simulink model "EPT"  (R2019b)
settings: Solver=FixedStepDiscrete  StartTime=0.0  StopTime=5  FixedStep=0.005  RelTol=1e-3  EnableMultiTasking=on
PreLoadFcn:
  | try, model_open; catch, disp('Error occurred while executing model pre-load callback: model_open.m'); disp('Please assure that the MATLAB working directory is set to the model directory before opening.'); end
InitFcn:
  | try, model_open; catch, end
undefined symbols (not defined in the file or in its folder): Bridge, GCM, H, ln, raptor_get_param_eval, raptor_get_safe_string, raptor_xcp_function
libraries: Raptor_lib x2810, simulink x374, hdlsllib x19
(part 22 of 45)

== system EPT/Foreground_TimeBase_5ms/CAN/CAN3_exec/SWCU/SWCU OP Status-G6 ==
  Trigger : TriggerPort  VariantControl=Variant  PortDimensions=1
  raptor_can_rxmsg : Raptor_lib/CAN/raptor_can_rxmsg  canDefinition=struct('dbcFile', 'EPTvsSWCU.dbc','message', 'SWCU_OP_Status_G6_SWUBP1','comment', '','signals', {{'SWCU_BPSWU_READY','SWCU_BPSWU_HV_ENABLED','SWCU_BPSWU_EW','SWCU_BPSWU_EW_CODE','SWCU_BPSWU_FCCAP','SWCU_BPSWU_RSOC','SWCU_BPSWU_CURR','SWCU_BPSWU_VOLT','SWCU_BPSWU_TEMP','SWCU_BPSWU_VCELL_MAX','SWCU_BPSWU_VCELL_MIN'}},'enabled', [ 1 1 1 1 1 1 1 1 1 1 1;],'canBus', '''CAN3''','messageID', [ 410055780;],'idMask', [ 536870911;],'payloadMask', [],'payloadValue', [],'period', [ 0;],'mailbox', '''''','queueSize', [ 1;],'label', [ 1;],'ver', [ 2;],'showID', [ 0;],'showRaw', [ 0;],'fill', [ 0;],'editID', [ 0;],'signalOrder', [ 2;])  canBus='CAN3'  mailbox=''  payloadMask=[]  payloadValue=[]  idMask=hex2dec('1FFFFFFF')  queueSize=1  showID=0  label=1  fill=0  id=410055780  showRaw=0  showAge=1  signalOrder=2  signalInfo={{struct('Name', 'SWCU_BPSWU_HV_ENABLED','Startbit', [ 0;],'SignalSize', [ 1;],'ByteOrder', 'LittleEndian','ValueType', 'UNSIGNED','Class', 'uint8','Signed', [ 0;],'Factor', [ 1;],'Offset', [ 0;],'Min', [ 0;],'Max', [ 0;],'Units', '','Comment', '','StartBit', [ 1;]),struct('Name', 'SWCU_BPSWU_EW_CODE','Startbit', [ 0;],'SignalSize', [ 5;],'ByteOrder', 'LittleEndian','ValueType', 'UNSIGNED','Class', 'uint8','Signed', [ 0;],'Factor', [ 1;],'Offset', [ 0;],'Min', [ 0;],'Max', [ 0;],'Units', '','Comment', '','StartBit', [ 3;]),struct('Name', 'SWCU_BPSWU_EW','Startbit', [ 0;],'SignalSize', [ 1;],'ByteOrder', 'LittleEndian','ValueType', 'UNSIGNED','Class', 'uint8','Signed', [ 0;],'Factor', [ 1;],'Offset', [ 0;],'Min', [ 0;],'Max', [ 0;],'Units', '','Comment', '','StartBit', [ 2;]),struct('Name', 'SWCU_BPSWU_VCELL_MIN','Startbit', [ 0;],'SignalSize', [ 8;],'ByteOrder', 'LittleEndian','ValueType', 'UNSIGNED','Class', 'uint8','Signed', [ 0;],'Factor', [ 0.01;],'Offset', [ 2;],'Min', [ 0;],'Max', [ 0;],'Units', 'V','Comment', '','StartBit', [ 56;]),struct('Name', 'SWCU_BPSWU_VCELL_MAX','Startbit', [ 0;],'SignalSize', [ 8;],'ByteOrder', 'LittleEndian','ValueType', 'UNSIGNED','Class', 'uint8','Signed', [ 0;],'Factor', [ 0.01;],'Offset', [ 2;],'Min', [ 0;],'Max', [ 0;],'Units', 'V','Comment', '','StartBit', [ 48;]),struct('Name', 'SWCU_BPSWU_VOLT','Startbit', [ 0;],'SignalSize', [ 8;],'ByteOrder', 'LittleEndian','ValueType', 'UNSIGNED','Class', 'uint8','Signed', [ 0;],'Factor', [ 1;],'Offset', [ 0;],'Min', [ 0;],'Max', [ 0;],'Units', 'V','Comment', '','StartBit', [ 32;]),struct('Name', 'SWCU_BPSWU_TEMP','Startbit', [ 0;],'SignalSize', [ 8;],'ByteOrder', 'LittleEndian','ValueType', 'UNSIGNED','Class', 'uint8','Signed', [ 0;],'Factor', [ 1;],'Offset', [ -40;],'Min', [ 0;],'Max', [ 0;],'Units', '℃','Comment', '','StartBit', [ 40;]),struct('Name', 'SWCU_BPSWU_RSOC','Startbit', [ 0;],'SignalSize', [ 8;],'ByteOrder', 'LittleEndian','ValueType', 'UNSIGNED','Class', 'uint8','Signed', [ 0;],'Factor', [ 0.5;],'Offset', [ -12.5;],'Min', [ 0;],'Max', [ 0;],'Units', '%','Comment', '','StartBit', [ 16;]),struct('Name', 'SWCU_BPSWU_CURR','Startbit', [ 0;],'SignalSize', [ 8;],'ByteOrder', 'LittleEndian','ValueType', 'UNSIGNED','Class', 'uint8','Signed', [ 0;],'Factor', [ 0.8;],'Offset', [ -100;],'Min', [ 0;],'Max', [ 0;],'Units', 'A','Comment', '','StartBit', [ 24;]),struct('Name', 'SWCU_BPSWU_FCCAP','Startbit', [ 0;],'SignalSize', [ 8;],'ByteOrder', 'LittleEndian','ValueType', 'UNSIGNED','Class', 'uint8','Signed', [ 0;],'Factor', [ 0.4;],'Offset', [ 0;],'Min', [ 0;],'Max', [ 0;],'Units', 'Ah','Comment', '','StartBit', [ 8;]),struct('Name', 'SWCU_BPSWU_READY','Startbit', [ 0;],'SignalSize', [ 1;],'ByteOrder', 'LittleEndian','ValueType', 'UNSIGNED','Class', 'uint8','Signed', [ 0;],'Factor', [ 1;],'Offset', [ 0;],'Min', [ 0;],'Max', [ 0;],'Units', '','Comment', '','StartBit', [ 0;])}}
      settings: SourceProductName=Raptor
  raptor_data_def : Raptor_lib/Data Storage/raptor_data_def  dataName='SWCU_BPSWU1_HV_ENABLED'  initValue=0  dataType=double  storage=Calibration  calVisible=on  calType=Measurement  calDispType=Number  calEnum={'False', 'True'}  calGain=1.0  calOffset=0  calMin=-inf  calMax=inf  calFormat='-1'  calUnit=''  calHelp=''  calAccess=1  calFunction=raptor_xcp_function(gcb)  calDispHeaders=off  calColHeaders={'Col1' 'Col2' 'Col3'}  calRowHeaders={'Row1' 'Row2' 'Row3'}
      settings: SourceProductName=Raptor
  raptor_data_def1 : Raptor_lib/Data Storage/raptor_data_def  dataName='SWCU_BPSWU1_READY'  initValue=0  dataType=double  storage=Calibration  calVisible=on  calType=Measurement  calDispType=Number  calEnum={'False', 'True'}  calGain=1.0  calOffset=0  calMin=-inf  calMax=inf  calFormat='-1'  calUnit=''  calHelp=''  calAccess=1  calFunction=raptor_xcp_function(gcb)  calDispHeaders=off  calColHeaders={'Col1' 'Col2' 'Col3'}  calRowHeaders={'Row1' 'Row2' 'Row3'}
      settings: SourceProductName=Raptor
  raptor_data_def10 : Raptor_lib/Data Storage/raptor_data_def  dataName='SWCU_BPSWU1_VCELL_MAX'  initValue=0  dataType=double  storage=Calibration  calVisible=on  calType=Measurement  calDispType=Number  calEnum={'False', 'True'}  calGain=1.0  calOffset=0  calMin=-inf  calMax=inf  calFormat='-1'  calUnit=''  calHelp=''  calAccess=1  calFunction=raptor_xcp_function(gcb)  calDispHeaders=off  calColHeaders={'Col1' 'Col2' 'Col3'}  calRowHeaders={'Row1' 'Row2' 'Row3'}
      settings: SourceProductName=Raptor
  raptor_data_def2 : Raptor_lib/Data Storage/raptor_data_def  dataName='SWCU_BPSWU1_EW'  initValue=0  dataType=double  storage=Calibration  calVisible=on  calType=Measurement  calDispType=Number  calEnum={'False', 'True'}  calGain=1.0  calOffset=0  calMin=-inf  calMax=inf  calFormat='-1'  calUnit=''  calHelp=''  calAccess=1  calFunction=raptor_xcp_function(gcb)  calDispHeaders=off  calColHeaders={'Col1' 'Col2' 'Col3'}  calRowHeaders={'Row1' 'Row2' 'Row3'}
      settings: SourceProductName=Raptor
  raptor_data_def3 : Raptor_lib/Data Storage/raptor_data_def  dataName='SWCU_BPSWU1_FCCAP'  initValue=0  dataType=double  storage=Calibration  calVisible=on  calType=Measurement  calDispType=Number  calEnum={'False', 'True'}  calGain=1.0  calOffset=0  calMin=-inf  calMax=inf  calFormat='-1'  calUnit=''  calHelp=''  calAccess=1  calFunction=raptor_xcp_function(gcb)  calDispHeaders=off  calColHeaders={'Col1' 'Col2' 'Col3'}  calRowHeaders={'Row1' 'Row2' 'Row3'}
      settings: SourceProductName=Raptor
  raptor_data_def4 : Raptor_lib/Data Storage/raptor_data_def  dataName='SWCU_BPSWU1_RSOC'  initValue=0  dataType=double  storage=Calibration  calVisible=on  calType=Measurement  calDispType=Number  calEnum={'False', 'True'}  calGain=1.0  calOffset=0  calMin=-inf  calMax=inf  calFormat='-1'  calUnit=''  calHelp=''  calAccess=1  calFunction=raptor_xcp_function(gcb)  calDispHeaders=off  calColHeaders={'Col1' 'Col2' 'Col3'}  calRowHeaders={'Row1' 'Row2' 'Row3'}
      settings: SourceProductName=Raptor
  raptor_data_def5 : Raptor_lib/Data Storage/raptor_data_def  dataName='SWCU_BPSWU1_EW_CODE'  initValue=0  dataType=double  storage=Calibration  calVisible=on  calType=Measurement  calDispType=Number  calEnum={'False', 'True'}  calGain=1.0  calOffset=0  calMin=-inf  calMax=inf  calFormat='-1'  calUnit=''  calHelp=''  calAccess=1  calFunction=raptor_xcp_function(gcb)  calDispHeaders=off  calColHeaders={'Col1' 'Col2' 'Col3'}  calRowHeaders={'Row1' 'Row2' 'Row3'}
      settings: SourceProductName=Raptor
  raptor_data_def6 : Raptor_lib/Data Storage/raptor_data_def  dataName='SWCU_BPSWU1_CURR'  initValue=0  dataType=double  storage=Calibration  calVisible=on  calType=Measurement  calDispType=Number  calEnum={'False', 'True'}  calGain=1.0  calOffset=0  calMin=-inf  calMax=inf  calFormat='-1'  calUnit=''  calHelp=''  calAccess=1  calFunction=raptor_xcp_function(gcb)  calDispHeaders=off  calColHeaders={'Col1' 'Col2' 'Col3'}  calRowHeaders={'Row1' 'Row2' 'Row3'}
      settings: SourceProductName=Raptor
  raptor_data_def7 : Raptor_lib/Data Storage/raptor_data_def  dataName='SWCU_BPSWU1_TEMP'  initValue=0  dataType=double  storage=Calibration  calVisible=on  calType=Measurement  calDispType=Number  calEnum={'False', 'True'}  calGain=1.0  calOffset=0  calMin=-inf  calMax=inf  calFormat='-1'  calUnit=''  calHelp=''  calAccess=1  calFunction=raptor_xcp_function(gcb)  calDispHeaders=off  calColHeaders={'Col1' 'Col2' 'Col3'}  calRowHeaders={'Row1' 'Row2' 'Row3'}
      settings: SourceProductName=Raptor
  raptor_data_def8 : Raptor_lib/Data Storage/raptor_data_def  dataName='SWCU_BPSWU1_VCELL_MIN'  initValue=0  dataType=double  storage=Calibration  calVisible=on  calType=Measurement  calDispType=Number  calEnum={'False', 'True'}  calGain=1.0  calOffset=0  calMin=-inf  calMax=inf  calFormat='-1'  calUnit=''  calHelp=''  calAccess=1  calFunction=raptor_xcp_function(gcb)  calDispHeaders=off  calColHeaders={'Col1' 'Col2' 'Col3'}  calRowHeaders={'Row1' 'Row2' 'Row3'}
      settings: SourceProductName=Raptor
  raptor_data_def9 : Raptor_lib/Data Storage/raptor_data_def  dataName='SWCU_BPSWU1_VOLT'  initValue=0  dataType=double  storage=Calibration  calVisible=on  calType=Measurement  calDispType=Number  calEnum={'False', 'True'}  calGain=1.0  calOffset=0  calMin=-inf  calMax=inf  calFormat='-1'  calUnit=''  calHelp=''  calAccess=1  calFunction=raptor_xcp_function(gcb)  calDispHeaders=off  calColHeaders={'Col1' 'Col2' 'Col3'}  calRowHeaders={'Row1' 'Row2' 'Row3'}
      settings: SourceProductName=Raptor
  raptor_data_write : Raptor_lib/Data Storage/raptor_data_write  dataName='SWCU_BPSWU1_HV_ENABLED'  dataShape=Scalar  idxSource=Input Port  idxRow=1  idxCol=1
      settings: SourceProductName=Raptor
  raptor_data_write1 : Raptor_lib/Data Storage/raptor_data_write  dataName='SWCU_BPSWU1_READY'  dataShape=Scalar  idxSource=Input Port  idxRow=1  idxCol=1
      settings: SourceProductName=Raptor
  raptor_data_write10 : Raptor_lib/Data Storage/raptor_data_write  dataName='SWCU_BPSWU1_VCELL_MIN'  dataShape=Scalar  idxSource=Input Port  idxRow=1  idxCol=1
      settings: SourceProductName=Raptor
  raptor_data_write2 : Raptor_lib/Data Storage/raptor_data_write  dataName='SWCU_BPSWU1_EW'  dataShape=Scalar  idxSource=Input Port  idxRow=1  idxCol=1
      settings: SourceProductName=Raptor
  raptor_data_write3 : Raptor_lib/Data Storage/raptor_data_write  dataName='SWCU_BPSWU1_EW_CODE'  dataShape=Scalar  idxSource=Input Port  idxRow=1  idxCol=1
      settings: SourceProductName=Raptor
  raptor_data_write4 : Raptor_lib/Data Storage/raptor_data_write  dataName='SWCU_BPSWU1_RSOC'  dataShape=Scalar  idxSource=Input Port  idxRow=1  idxCol=1
      settings: SourceProductName=Raptor
  raptor_data_write5 : Raptor_lib/Data Storage/raptor_data_write  dataName='SWCU_BPSWU1_FCCAP'  dataShape=Scalar  idxSource=Input Port  idxRow=1  idxCol=1
      settings: SourceProductName=Raptor
  raptor_data_write6 : Raptor_lib/Data Storage/raptor_data_write  dataName='SWCU_BPSWU1_CURR'  dataShape=Scalar  idxSource=Input Port  idxRow=1  idxCol=1
      settings: SourceProductName=Raptor
  raptor_data_write7 : Raptor_lib/Data Storage/raptor_data_write  dataName='SWCU_BPSWU1_VOLT'  dataShape=Scalar  idxSource=Input Port  idxRow=1  idxCol=1
      settings: SourceProductName=Raptor
  raptor_data_write8 : Raptor_lib/Data Storage/raptor_data_write  dataName='SWCU_BPSWU1_TEMP'  dataShape=Scalar  idxSource=Input Port  idxRow=1  idxCol=1
      settings: SourceProductName=Raptor
  raptor_data_write9 : Raptor_lib/Data Storage/raptor_data_write  dataName='SWCU_BPSWU1_VCELL_MAX'  dataShape=Scalar  idxSource=Input Port  idxRow=1  idxCol=1
      settings: SourceProductName=Raptor
  wires:
  raptor_can_rxmsg/3 -> raptor_data_write/1  "SWCU_BPSWU_HV_ENABLED"
  raptor_can_rxmsg/2 -> raptor_data_write1/1  "SWCU_BPSWU_READY"
  raptor_can_rxmsg/4 -> raptor_data_write2/1  "SWCU_BPSWU_EW"
  raptor_can_rxmsg/5 -> raptor_data_write3/1  "SWCU_BPSWU_EW_CODE"
  raptor_can_rxmsg/9 -> raptor_data_write7/1  "SWCU_BPSWU_VOLT"
  raptor_can_rxmsg/8 -> raptor_data_write6/1  "SWCU_BPSWU_CURR"
  raptor_can_rxmsg/6 -> raptor_data_write5/1  "SWCU_BPSWU_FCCAP"
  raptor_can_rxmsg/7 -> raptor_data_write4/1  "SWCU_BPSWU_RSOC"
  raptor_can_rxmsg/10 -> raptor_data_write8/1  "SWCU_BPSWU_TEMP"
  raptor_can_rxmsg/11 -> raptor_data_write9/1  "SWCU_BPSWU_VCELL_MAX"
  raptor_can_rxmsg/12 -> raptor_data_write10/1  "SWCU_BPSWU_VCELL_MIN"

== system EPT/Foreground_TimeBase_5ms/CAN/CAN3_exec/SWCU/SWCU OP Status-G7 ==
  Trigger : TriggerPort  VariantControl=Variant  PortDimensions=1
  raptor_can_rxmsg : Raptor_lib/CAN/raptor_can_rxmsg  canDefinition=struct('dbcFile', 'EPTvsSWCU.dbc','message', 'SWCU_OP_Status_G7_SWUBP2','comment', '','signals', {{'SWCU_BPSWU_READY','SWCU_BPSWU_HV_ENABLED','SWCU_BPSWU_EW','SWCU_BPSWU_EW_CODE','SWCU_BPSWU_FCCAP','SWCU_BPSWU_RSOC','SWCU_BPSWU_CURR','SWCU_BPSWU_VOLT','SWCU_BPSWU_TEMP','SWCU_BPSWU_VCELL_MAX','SWCU_BPSWU_VCELL_MIN'}},'enabled', [ 1 1 1 1 1 1 1 1 1 1 1;],'canBus', '''CAN3''','messageID', [ 410121316;],'idMask', [ 536870911;],'payloadMask', [],'payloadValue', [],'period', [ 0;],'mailbox', '''''','queueSize', [ 1;],'label', [ 0;],'ver', [ 2;],'showID', [ 0;],'showRaw', [ 0;],'fill', [ 0;],'editID', [ 0;],'signalOrder', [ 2;])  canBus='CAN3'  mailbox=''  payloadMask=[]  payloadValue=[]  idMask=hex2dec('1FFFFFFF')  queueSize=1  showID=0  label=0  fill=0  id=410121316  showRaw=0  showAge=1  signalOrder=2  signalInfo={{struct('Name', 'SWCU_BPSWU_HV_ENABLED','Startbit', [ 0;],'SignalSize', [ 1;],'ByteOrder', 'LittleEndian','ValueType', 'UNSIGNED','Class', 'uint8','Signed', [ 0;],'Factor', [ 1;],'Offset', [ 0;],'Min', [ 0;],'Max', [ 0;],'Units', '','Comment', '','StartBit', [ 1;]),struct('Name', 'SWCU_BPSWU_EW_CODE','Startbit', [ 0;],'SignalSize', [ 5;],'ByteOrder', 'LittleEndian','ValueType', 'UNSIGNED','Class', 'uint8','Signed', [ 0;],'Factor', [ 1;],'Offset', [ 0;],'Min', [ 0;],'Max', [ 0;],'Units', '','Comment', '','StartBit', [ 3;]),struct('Name', 'SWCU_BPSWU_EW','Startbit', [ 0;],'SignalSize', [ 1;],'ByteOrder', 'LittleEndian','ValueType', 'UNSIGNED','Class', 'uint8','Signed', [ 0;],'Factor', [ 1;],'Offset', [ 0;],'Min', [ 0;],'Max', [ 0;],'Units', '','Comment', '','StartBit', [ 2;]),struct('Name', 'SWCU_BPSWU_VCELL_MIN','Startbit', [ 0;],'SignalSize', [ 8;],'ByteOrder', 'LittleEndian','ValueType', 'UNSIGNED','Class', 'uint8','Signed', [ 0;],'Factor', [ 0.01;],'Offset', [ 2;],'Min', [ 0;],'Max', [ 0;],'Units', 'V','Comment', '','StartBit', [ 56;]),struct('Name', 'SWCU_BPSWU_VCELL_MAX','Startbit', [ 0;],'SignalSize', [ 8;],'ByteOrder', 'LittleEndian','ValueType', 'UNSIGNED','Class', 'uint8','Signed', [ 0;],'Factor', [ 0.01;],'Offset', [ 2;],'Min', [ 0;],'Max', [ 0;],'Units', 'V','Comment', '','StartBit', [ 48;]),struct('Name', 'SWCU_BPSWU_VOLT','Startbit', [ 0;],'SignalSize', [ 8;],'ByteOrder', 'LittleEndian','ValueType', 'UNSIGNED','Class', 'uint8','Signed', [ 0;],'Factor', [ 1;],'Offset', [ 0;],'Min', [ 0;],'Max', [ 0;],'Units', 'V','Comment', '','StartBit', [ 32;]),struct('Name', 'SWCU_BPSWU_TEMP','Startbit', [ 0;],'SignalSize', [ 8;],'ByteOrder', 'LittleEndian','ValueType', 'UNSIGNED','Class', 'uint8','Signed', [ 0;],'Factor', [ 1;],'Offset', [ -40;],'Min', [ 0;],'Max', [ 0;],'Units', '℃','Comment', '','StartBit', [ 40;]),struct('Name', 'SWCU_BPSWU_RSOC','Startbit', [ 0;],'SignalSize', [ 8;],'ByteOrder', 'LittleEndian','ValueType', 'UNSIGNED','Class', 'uint8','Signed', [ 0;],'Factor', [ 0.5;],'Offset', [ -12.5;],'Min', [ 0;],'Max', [ 0;],'Units', '%','Comment', '','StartBit', [ 16;]),struct('Name', 'SWCU_BPSWU_CURR','Startbit', [ 0;],'SignalSize', [ 8;],'ByteOrder', 'LittleEndian','ValueType', 'UNSIGNED','Class', 'uint8','Signed', [ 0;],'Factor', [ 0.8;],'Offset', [ -100;],'Min', [ 0;],'Max', [ 0;],'Units', 'A','Comment', '','StartBit', [ 24;]),struct('Name', 'SWCU_BPSWU_FCCAP','Startbit', [ 0;],'SignalSize', [ 8;],'ByteOrder', 'LittleEndian','ValueType', 'UNSIGNED','Class', 'uint8','Signed', [ 0;],'Factor', [ 0.4;],'Offset', [ 0;],'Min', [ 0;],'Max', [ 0;],'Units', 'Ah','Comment', '','StartBit', [ 8;]),struct('Name', 'SWCU_BPSWU_READY','Startbit', [ 0;],'SignalSize', [ 1;],'ByteOrder', 'LittleEndian','ValueType', 'UNSIGNED','Class', 'uint8','Signed', [ 0;],'Factor', [ 1;],'Offset', [ 0;],'Min', [ 0;],'Max', [ 0;],'Units', '','Comment', '','StartBit', [ 0;])}}
      settings: SourceProductName=Raptor
  raptor_data_def : Raptor_lib/Data Storage/raptor_data_def  dataName='SWCU_BPSWU2_HV_ENABLED'  initValue=0  dataType=double  storage=Calibration  calVisible=on  calType=Measurement  calDispType=Number  calEnum={'False', 'True'}  calGain=1.0  calOffset=0  calMin=-inf  calMax=inf  calFormat='-1'  calUnit=''  calHelp=''  calAccess=1  calFunction=raptor_xcp_function(gcb)  calDispHeaders=off  calColHeaders={'Col1' 'Col2' 'Col3'}  calRowHeaders={'Row1' 'Row2' 'Row3'}
      settings: SourceProductName=Raptor
  raptor_data_def1 : Raptor_lib/Data Storage/raptor_data_def  dataName='SWCU_BPSWU2_READY'  initValue=0  dataType=double  storage=Calibration  calVisible=on  calType=Measurement  calDispType=Number  calEnum={'False', 'True'}  calGain=1.0  calOffset=0  calMin=-inf  calMax=inf  calFormat='-1'  calUnit=''  calHelp=''  calAccess=1  calFunction=raptor_xcp_function(gcb)  calDispHeaders=off  calColHeaders={'Col1' 'Col2' 'Col3'}  calRowHeaders={'Row1' 'Row2' 'Row3'}
      settings: SourceProductName=Raptor
  raptor_data_def10 : Raptor_lib/Data Storage/raptor_data_def  dataName='SWCU_BPSWU2_VCELL_MAX'  initValue=0  dataType=double  storage=Calibration  calVisible=on  calType=Measurement  calDispType=Number  calEnum={'False', 'True'}  calGain=1.0  calOffset=0  calMin=-inf  calMax=inf  calFormat='-1'  calUnit=''  calHelp=''  calAccess=1  calFunction=raptor_xcp_function(gcb)  calDispHeaders=off  calColHeaders={'Col1' 'Col2' 'Col3'}  calRowHeaders={'Row1' 'Row2' 'Row3'}
      settings: SourceProductName=Raptor
  raptor_data_def2 : Raptor_lib/Data Storage/raptor_data_def  dataName='SWCU_BPSWU2_EW'  initValue=0  dataType=double  storage=Calibration  calVisible=on  calType=Measurement  calDispType=Number  calEnum={'False', 'True'}  calGain=1.0  calOffset=0  calMin=-inf  calMax=inf  calFormat='-1'  calUnit=''  calHelp=''  calAccess=1  calFunction=raptor_xcp_function(gcb)  calDispHeaders=off  calColHeaders={'Col1' 'Col2' 'Col3'}  calRowHeaders={'Row1' 'Row2' 'Row3'}
      settings: SourceProductName=Raptor
  raptor_data_def3 : Raptor_lib/Data Storage/raptor_data_def  dataName='SWCU_BPSWU2_FCCAP'  initValue=0  dataType=double  storage=Calibration  calVisible=on  calType=Measurement  calDispType=Number  calEnum={'False', 'True'}  calGain=1.0  calOffset=0  calMin=-inf  calMax=inf  calFormat='-1'  calUnit=''  calHelp=''  calAccess=1  calFunction=raptor_xcp_function(gcb)  calDispHeaders=off  calColHeaders={'Col1' 'Col2' 'Col3'}  calRowHeaders={'Row1' 'Row2' 'Row3'}
      settings: SourceProductName=Raptor
  raptor_data_def4 : Raptor_lib/Data Storage/raptor_data_def  dataName='SWCU_BPSWU2_RSOC'  initValue=0  dataType=double  storage=Calibration  calVisible=on  calType=Measurement  calDispType=Number  calEnum={'False', 'True'}  calGain=1.0  calOffset=0  calMin=-inf  calMax=inf  calFormat='-1'  calUnit=''  calHelp=''  calAccess=1  calFunction=raptor_xcp_function(gcb)  calDispHeaders=off  calColHeaders={'Col1' 'Col2' 'Col3'}  calRowHeaders={'Row1' 'Row2' 'Row3'}
      settings: SourceProductName=Raptor
  raptor_data_def5 : Raptor_lib/Data Storage/raptor_data_def  dataName='SWCU_BPSWU2_EW_CODE'  initValue=0  dataType=double  storage=Calibration  calVisible=on  calType=Measurement  calDispType=Number  calEnum={'False', 'True'}  calGain=1.0  calOffset=0  calMin=-inf  calMax=inf  calFormat='-1'  calUnit=''  calHelp=''  calAccess=1  calFunction=raptor_xcp_function(gcb)  calDispHeaders=off  calColHeaders={'Col1' 'Col2' 'Col3'}  calRowHeaders={'Row1' 'Row2' 'Row3'}
      settings: SourceProductName=Raptor
  raptor_data_def6 : Raptor_lib/Data Storage/raptor_data_def  dataName='SWCU_BPSWU2_CURR'  initValue=0  dataType=double  storage=Calibration  calVisible=on  calType=Measurement  calDispType=Number  calEnum={'False', 'True'}  calGain=1.0  calOffset=0  calMin=-inf  calMax=inf  calFormat='-1'  calUnit=''  calHelp=''  calAccess=1  calFunction=raptor_xcp_function(gcb)  calDispHeaders=off  calColHeaders={'Col1' 'Col2' 'Col3'}  calRowHeaders={'Row1' 'Row2' 'Row3'}
      settings: SourceProductName=Raptor
  raptor_data_def7 : Raptor_lib/Data Storage/raptor_data_def  dataName='SWCU_BPSWU2_TEMP'  initValue=0  dataType=double  storage=Calibration  calVisible=on  calType=Measurement  calDispType=Number  calEnum={'False', 'True'}  calGain=1.0  calOffset=0  calMin=-inf  calMax=inf  calFormat='-1'  calUnit=''  calHelp=''  calAccess=1  calFunction=raptor_xcp_function(gcb)  calDispHeaders=off  calColHeaders={'Col1' 'Col2' 'Col3'}  calRowHeaders={'Row1' 'Row2' 'Row3'}
      settings: SourceProductName=Raptor
  raptor_data_def8 : Raptor_lib/Data Storage/raptor_data_def  dataName='SWCU_BPSWU2_VCELL_MIN'  initValue=0  dataType=double  storage=Calibration  calVisible=on  calType=Measurement  calDispType=Number  calEnum={'False', 'True'}  calGain=1.0  calOffset=0  calMin=-inf  calMax=inf  calFormat='-1'  calUnit=''  calHelp=''  calAccess=1  calFunction=raptor_xcp_function(gcb)  calDispHeaders=off  calColHeaders={'Col1' 'Col2' 'Col3'}  calRowHeaders={'Row1' 'Row2' 'Row3'}
      settings: SourceProductName=Raptor
  raptor_data_def9 : Raptor_lib/Data Storage/raptor_data_def  dataName='SWCU_BPSWU2_VOLT'  initValue=0  dataType=double  storage=Calibration  calVisible=on  calType=Measurement  calDispType=Number  calEnum={'False', 'True'}  calGain=1.0  calOffset=0  calMin=-inf  calMax=inf  calFormat='-1'  calUnit=''  calHelp=''  calAccess=1  calFunction=raptor_xcp_function(gcb)  calDispHeaders=off  calColHeaders={'Col1' 'Col2' 'Col3'}  calRowHeaders={'Row1' 'Row2' 'Row3'}
      settings: SourceProductName=Raptor
  raptor_data_write : Raptor_lib/Data Storage/raptor_data_write  dataName='SWCU_BPSWU2_HV_ENABLED'  dataShape=Scalar  idxSource=Input Port  idxRow=1  idxCol=1
      settings: SourceProductName=Raptor
  raptor_data_write1 : Raptor_lib/Data Storage/raptor_data_write  dataName='SWCU_BPSWU2_READY'  dataShape=Scalar  idxSource=Input Port  idxRow=1  idxCol=1
      settings: SourceProductName=Raptor
  raptor_data_write10 : Raptor_lib/Data Storage/raptor_data_write  dataName='SWCU_BPSWU2_VCELL_MIN'  dataShape=Scalar  idxSource=Input Port  idxRow=1  idxCol=1
      settings: SourceProductName=Raptor
  raptor_data_write2 : Raptor_lib/Data Storage/raptor_data_write  dataName='SWCU_BPSWU2_EW'  dataShape=Scalar  idxSource=Input Port  idxRow=1  idxCol=1
      settings: SourceProductName=Raptor
  raptor_data_write3 : Raptor_lib/Data Storage/raptor_data_write  dataName='SWCU_BPSWU2_EW_CODE'  dataShape=Scalar  idxSource=Input Port  idxRow=1  idxCol=1
      settings: SourceProductName=Raptor
  raptor_data_write4 : Raptor_lib/Data Storage/raptor_data_write  dataName='SWCU_BPSWU2_RSOC'  dataShape=Scalar  idxSource=Input Port  idxRow=1  idxCol=1
      settings: SourceProductName=Raptor
  raptor_data_write5 : Raptor_lib/Data Storage/raptor_data_write  dataName='SWCU_BPSWU2_FCCAP'  dataShape=Scalar  idxSource=Input Port  idxRow=1  idxCol=1
      settings: SourceProductName=Raptor
  raptor_data_write6 : Raptor_lib/Data Storage/raptor_data_write  dataName='SWCU_BPSWU2_CURR'  dataShape=Scalar  idxSource=Input Port  idxRow=1  idxCol=1
      settings: SourceProductName=Raptor
  raptor_data_write7 : Raptor_lib/Data Storage/raptor_data_write  dataName='SWCU_BPSWU2_VOLT'  dataShape=Scalar  idxSource=Input Port  idxRow=1  idxCol=1
      settings: SourceProductName=Raptor
  raptor_data_write8 : Raptor_lib/Data Storage/raptor_data_write  dataName='SWCU_BPSWU2_TEMP'  dataShape=Scalar  idxSource=Input Port  idxRow=1  idxCol=1
      settings: SourceProductName=Raptor
  raptor_data_write9 : Raptor_lib/Data Storage/raptor_data_write  dataName='SWCU_BPSWU2_VCELL_MAX'  dataShape=Scalar  idxSource=Input Port  idxRow=1  idxCol=1
      settings: SourceProductName=Raptor
  wires:
  raptor_can_rxmsg/3 -> raptor_data_write/1  "SWCU_BPSWU_HV_ENABLED"
  raptor_can_rxmsg/8 -> raptor_data_write6/1  "SWCU_BPSWU_CURR"
  raptor_can_rxmsg/6 -> raptor_data_write5/1  "SWCU_BPSWU_FCCAP"
  raptor_can_rxmsg/9 -> raptor_data_write7/1  "SWCU_BPSWU_VOLT"
  raptor_can_rxmsg/7 -> raptor_data_write4/1  "SWCU_BPSWU_RSOC"
  raptor_can_rxmsg/5 -> raptor_data_write3/1  "SWCU_BPSWU_EW_CODE"
  raptor_can_rxmsg/4 -> raptor_data_write2/1  "SWCU_BPSWU_EW"
  raptor_can_rxmsg/11 -> raptor_data_write9/1  "SWCU_BPSWU_VCELL_MAX"
  raptor_can_rxmsg/12 -> raptor_data_write10/1  "SWCU_BPSWU_VCELL_MIN"
  raptor_can_rxmsg/2 -> raptor_data_write1/1  "SWCU_BPSWU_READY"
  raptor_can_rxmsg/10 -> raptor_data_write8/1  "SWCU_BPSWU_TEMP"

== system EPT/Foreground_TimeBase_5ms/CAN/CAN3_exec/SWCU/SWCU OP Status-G8 ==
  Trigger : TriggerPort  VariantControl=Variant  PortDimensions=1
  raptor_can_rxmsg : Raptor_lib/CAN/raptor_can_rxmsg  canDefinition=struct('dbcFile', 'EPTvsSWCU.dbc','message', 'SWCU_OP_Status_G8_SWUBP3','comment', '','signals', {{'SWCU_BPSWU_READY','SWCU_BPSWU_HV_ENABLED','SWCU_BPSWU_EW','SWCU_BPSWU_EW_CODE','SWCU_BPSWU_FCCAP','SWCU_BPSWU_RSOC','SWCU_BPSWU_CURR','SWCU_BPSWU_VOLT','SWCU_BPSWU_TEMP','SWCU_BPSWU_VCELL_MAX','SWCU_BPSWU_VCELL_MIN'}},'enabled', [ 1 1 1 1 1 1 1 1 1 1 1;],'canBus', '''CAN3''','messageID', [ 410186852;],'idMask', [ 536870911;],'payloadMask', [],'payloadValue', [],'period', [ 0;],'mailbox', '''''','queueSize', [ 1;],'label', [ 0;],'ver', [ 2;],'showID', [ 0;],'showRaw', [ 0;],'fill', [ 0;],'editID', [ 0;],'signalOrder', [ 2;])  canBus='CAN3'  mailbox=''  payloadMask=[]  payloadValue=[]  idMask=hex2dec('1FFFFFFF')  queueSize=1  showID=0  label=0  fill=0  id=410186852  showRaw=0  showAge=1  signalOrder=2  signalInfo={{struct('Name', 'SWCU_BPSWU_HV_ENABLED','Startbit', [ 0;],'SignalSize', [ 1;],'ByteOrder', 'LittleEndian','ValueType', 'UNSIGNED','Class', 'uint8','Signed', [ 0;],'Factor', [ 1;],'Offset', [ 0;],'Min', [ 0;],'Max', [ 0;],'Units', '','Comment', '','StartBit', [ 1;]),struct('Name', 'SWCU_BPSWU_EW_CODE','Startbit', [ 0;],'SignalSize', [ 5;],'ByteOrder', 'LittleEndian','ValueType', 'UNSIGNED','Class', 'uint8','Signed', [ 0;],'Factor', [ 1;],'Offset', [ 0;],'Min', [ 0;],'Max', [ 0;],'Units', '','Comment', '','StartBit', [ 3;]),struct('Name', 'SWCU_BPSWU_EW','Startbit', [ 0;],'SignalSize', [ 1;],'ByteOrder', 'LittleEndian','ValueType', 'UNSIGNED','Class', 'uint8','Signed', [ 0;],'Factor', [ 1;],'Offset', [ 0;],'Min', [ 0;],'Max', [ 0;],'Units', '','Comment', '','StartBit', [ 2;]),struct('Name', 'SWCU_BPSWU_VCELL_MIN','Startbit', [ 0;],'SignalSize', [ 8;],'ByteOrder', 'LittleEndian','ValueType', 'UNSIGNED','Class', 'uint8','Signed', [ 0;],'Factor', [ 0.01;],'Offset', [ 2;],'Min', [ 0;],'Max', [ 0;],'Units', 'V','Comment', '','StartBit', [ 56;]),struct('Name', 'SWCU_BPSWU_VCELL_MAX','Startbit', [ 0;],'SignalSize', [ 8;],'ByteOrder', 'LittleEndian','ValueType', 'UNSIGNED','Class', 'uint8','Signed', [ 0;],'Factor', [ 0.01;],'Offset', [ 2;],'Min', [ 0;],'Max', [ 0;],'Units', 'V','Comment', '','StartBit', [ 48;]),struct('Name', 'SWCU_BPSWU_VOLT','Startbit', [ 0;],'SignalSize', [ 8;],'ByteOrder', 'LittleEndian','ValueType', 'UNSIGNED','Class', 'uint8','Signed', [ 0;],'Factor', [ 1;],'Offset', [ 0;],'Min', [ 0;],'Max', [ 0;],'Units', 'V','Comment', '','StartBit', [ 32;]),struct('Name', 'SWCU_BPSWU_TEMP','Startbit', [ 0;],'SignalSize', [ 8;],'ByteOrder', 'LittleEndian','ValueType', 'UNSIGNED','Class', 'uint8','Signed', [ 0;],'Factor', [ 1;],'Offset', [ -40;],'Min', [ 0;],'Max', [ 0;],'Units', '℃','Comment', '','StartBit', [ 40;]),struct('Name', 'SWCU_BPSWU_RSOC','Startbit', [ 0;],'SignalSize', [ 8;],'ByteOrder', 'LittleEndian','ValueType', 'UNSIGNED','Class', 'uint8','Signed', [ 0;],'Factor', [ 0.5;],'Offset', [ -12.5;],'Min', [ 0;],'Max', [ 0;],'Units', '%','Comment', '','StartBit', [ 16;]),struct('Name', 'SWCU_BPSWU_CURR','Startbit', [ 0;],'SignalSize', [ 8;],'ByteOrder', 'LittleEndian','ValueType', 'UNSIGNED','Class', 'uint8','Signed', [ 0;],'Factor', [ 0.8;],'Offset', [ -100;],'Min', [ 0;],'Max', [ 0;],'Units', 'A','Comment', '','StartBit', [ 24;]),struct('Name', 'SWCU_BPSWU_FCCAP','Startbit', [ 0;],'SignalSize', [ 8;],'ByteOrder', 'LittleEndian','ValueType', 'UNSIGNED','Class', 'uint8','Signed', [ 0;],'Factor', [ 0.4;],'Offset', [ 0;],'Min', [ 0;],'Max', [ 0;],'Units', 'Ah','Comment', '','StartBit', [ 8;]),struct('Name', 'SWCU_BPSWU_READY','Startbit', [ 0;],'SignalSize', [ 1;],'ByteOrder', 'LittleEndian','ValueType', 'UNSIGNED','Class', 'uint8','Signed', [ 0;],'Factor', [ 1;],'Offset', [ 0;],'Min', [ 0;],'Max', [ 0;],'Units', '','Comment', '','StartBit', [ 0;])}}
      settings: SourceProductName=Raptor
  raptor_data_def : Raptor_lib/Data Storage/raptor_data_def  dataName='SWCU_BPSWU3_HV_ENABLED'  initValue=0  dataType=double  storage=Calibration  calVisible=on  calType=Measurement  calDispType=Number  calEnum={'False', 'True'}  calGain=1.0  calOffset=0  calMin=-inf  calMax=inf  calFormat='-1'  calUnit=''  calHelp=''  calAccess=1  calFunction=raptor_xcp_function(gcb)  calDispHeaders=off  calColHeaders={'Col1' 'Col2' 'Col3'}  calRowHeaders={'Row1' 'Row2' 'Row3'}
      settings: SourceProductName=Raptor
  raptor_data_def1 : Raptor_lib/Data Storage/raptor_data_def  dataName='SWCU_BPSWU3_READY'  initValue=0  dataType=double  storage=Calibration  calVisible=on  calType=Measurement  calDispType=Number  calEnum={'False', 'True'}  calGain=1.0  calOffset=0  calMin=-inf  calMax=inf  calFormat='-1'  calUnit=''  calHelp=''  calAccess=1  calFunction=raptor_xcp_function(gcb)  calDispHeaders=off  calColHeaders={'Col1' 'Col2' 'Col3'}  calRowHeaders={'Row1' 'Row2' 'Row3'}
      settings: SourceProductName=Raptor
  raptor_data_def10 : Raptor_lib/Data Storage/raptor_data_def  dataName='SWCU_BPSWU3_VCELL_MAX'  initValue=0  dataType=double  storage=Calibration  calVisible=on  calType=Measurement  calDispType=Number  calEnum={'False', 'True'}  calGain=1.0  calOffset=0  calMin=-inf  calMax=inf  calFormat='-1'  calUnit=''  calHelp=''  calAccess=1  calFunction=raptor_xcp_function(gcb)  calDispHeaders=off  calColHeaders={'Col1' 'Col2' 'Col3'}  calRowHeaders={'Row1' 'Row2' 'Row3'}
      settings: SourceProductName=Raptor
  raptor_data_def2 : Raptor_lib/Data Storage/raptor_data_def  dataName='SWCU_BPSWU3_EW'  initValue=0  dataType=double  storage=Calibration  calVisible=on  calType=Measurement  calDispType=Number  calEnum={'False', 'True'}  calGain=1.0  calOffset=0  calMin=-inf  calMax=inf  calFormat='-1'  calUnit=''  calHelp=''  calAccess=1  calFunction=raptor_xcp_function(gcb)  calDispHeaders=off  calColHeaders={'Col1' 'Col2' 'Col3'}  calRowHeaders={'Row1' 'Row2' 'Row3'}
      settings: SourceProductName=Raptor
  raptor_data_def3 : Raptor_lib/Data Storage/raptor_data_def  dataName='SWCU_BPSWU3_FCCAP'  initValue=0  dataType=double  storage=Calibration  calVisible=on  calType=Measurement  calDispType=Number  calEnum={'False', 'True'}  calGain=1.0  calOffset=0  calMin=-inf  calMax=inf  calFormat='-1'  calUnit=''  calHelp=''  calAccess=1  calFunction=raptor_xcp_function(gcb)  calDispHeaders=off  calColHeaders={'Col1' 'Col2' 'Col3'}  calRowHeaders={'Row1' 'Row2' 'Row3'}
      settings: SourceProductName=Raptor
  raptor_data_def4 : Raptor_lib/Data Storage/raptor_data_def  dataName='SWCU_BPSWU3_RSOC'  initValue=0  dataType=double  storage=Calibration  calVisible=on  calType=Measurement  calDispType=Number  calEnum={'False', 'True'}  calGain=1.0  calOffset=0  calMin=-inf  calMax=inf  calFormat='-1'  calUnit=''  calHelp=''  calAccess=1  calFunction=raptor_xcp_function(gcb)  calDispHeaders=off  calColHeaders={'Col1' 'Col2' 'Col3'}  calRowHeaders={'Row1' 'Row2' 'Row3'}
      settings: SourceProductName=Raptor
  raptor_data_def5 : Raptor_lib/Data Storage/raptor_data_def  dataName='SWCU_BPSWU3_EW_CODE'  initValue=0  dataType=double  storage=Calibration  calVisible=on  calType=Measurement  calDispType=Number  calEnum={'False', 'True'}  calGain=1.0  calOffset=0  calMin=-inf  calMax=inf  calFormat='-1'  calUnit=''  calHelp=''  calAccess=1  calFunction=raptor_xcp_function(gcb)  calDispHeaders=off  calColHeaders={'Col1' 'Col2' 'Col3'}  calRowHeaders={'Row1' 'Row2' 'Row3'}
      settings: SourceProductName=Raptor
  raptor_data_def6 : Raptor_lib/Data Storage/raptor_data_def  dataName='SWCU_BPSWU3_CURR'  initValue=0  dataType=double  storage=Calibration  calVisible=on  calType=Measurement  calDispType=Number  calEnum={'False', 'True'}  calGain=1.0  calOffset=0  calMin=-inf  calMax=inf  calFormat='-1'  calUnit=''  calHelp=''  calAccess=1  calFunction=raptor_xcp_function(gcb)  calDispHeaders=off  calColHeaders={'Col1' 'Col2' 'Col3'}  calRowHeaders={'Row1' 'Row2' 'Row3'}
      settings: SourceProductName=Raptor
  raptor_data_def7 : Raptor_lib/Data Storage/raptor_data_def  dataName='SWCU_BPSWU3_TEMP'  initValue=0  dataType=double  storage=Calibration  calVisible=on  calType=Measurement  calDispType=Number  calEnum={'False', 'True'}  calGain=1.0  calOffset=0  calMin=-inf  calMax=inf  calFormat='-1'  calUnit=''  calHelp=''  calAccess=1  calFunction=raptor_xcp_function(gcb)  calDispHeaders=off  calColHeaders={'Col1' 'Col2' 'Col3'}  calRowHeaders={'Row1' 'Row2' 'Row3'}
      settings: SourceProductName=Raptor
  raptor_data_def8 : Raptor_lib/Data Storage/raptor_data_def  dataName='SWCU_BPSWU3_VCELL_MIN'  initValue=0  dataType=double  storage=Calibration  calVisible=on  calType=Measurement  calDispType=Number  calEnum={'False', 'True'}  calGain=1.0  calOffset=0  calMin=-inf  calMax=inf  calFormat='-1'  calUnit=''  calHelp=''  calAccess=1  calFunction=raptor_xcp_function(gcb)  calDispHeaders=off  calColHeaders={'Col1' 'Col2' 'Col3'}  calRowHeaders={'Row1' 'Row2' 'Row3'}
      settings: SourceProductName=Raptor
  raptor_data_def9 : Raptor_lib/Data Storage/raptor_data_def  dataName='SWCU_BPSWU3_VOLT'  initValue=0  dataType=double  storage=Calibration  calVisible=on  calType=Measurement  calDispType=Number  calEnum={'False', 'True'}  calGain=1.0  calOffset=0  calMin=-inf  calMax=inf  calFormat='-1'  calUnit=''  calHelp=''  calAccess=1  calFunction=raptor_xcp_function(gcb)  calDispHeaders=off  calColHeaders={'Col1' 'Col2' 'Col3'}  calRowHeaders={'Row1' 'Row2' 'Row3'}
      settings: SourceProductName=Raptor
  raptor_data_write : Raptor_lib/Data Storage/raptor_data_write  dataName='SWCU_BPSWU3_HV_ENABLED'  dataShape=Scalar  idxSource=Input Port  idxRow=1  idxCol=1
      settings: SourceProductName=Raptor
  raptor_data_write1 : Raptor_lib/Data Storage/raptor_data_write  dataName='SWCU_BPSWU3_READY'  dataShape=Scalar  idxSource=Input Port  idxRow=1  idxCol=1
      settings: SourceProductName=Raptor
  raptor_data_write10 : Raptor_lib/Data Storage/raptor_data_write  dataName='SWCU_BPSWU3_VCELL_MIN'  dataShape=Scalar  idxSource=Input Port  idxRow=1  idxCol=1
      settings: SourceProductName=Raptor
  raptor_data_write2 : Raptor_lib/Data Storage/raptor_data_write  dataName='SWCU_BPSWU3_EW'  dataShape=Scalar  idxSource=Input Port  idxRow=1  idxCol=1
      settings: SourceProductName=Raptor
  raptor_data_write3 : Raptor_lib/Data Storage/raptor_data_write  dataName='SWCU_BPSWU3_EW_CODE'  dataShape=Scalar  idxSource=Input Port  idxRow=1  idxCol=1
      settings: SourceProductName=Raptor
  raptor_data_write4 : Raptor_lib/Data Storage/raptor_data_write  dataName='SWCU_BPSWU3_RSOC'  dataShape=Scalar  idxSource=Input Port  idxRow=1  idxCol=1
      settings: SourceProductName=Raptor
  raptor_data_write5 : Raptor_lib/Data Storage/raptor_data_write  dataName='SWCU_BPSWU3_FCCAP'  dataShape=Scalar  idxSource=Input Port  idxRow=1  idxCol=1
      settings: SourceProductName=Raptor
  raptor_data_write6 : Raptor_lib/Data Storage/raptor_data_write  dataName='SWCU_BPSWU3_CURR'  dataShape=Scalar  idxSource=Input Port  idxRow=1  idxCol=1
      settings: SourceProductName=Raptor
  raptor_data_write7 : Raptor_lib/Data Storage/raptor_data_write  dataName='SWCU_BPSWU3_VOLT'  dataShape=Scalar  idxSource=Input Port  idxRow=1  idxCol=1
      settings: SourceProductName=Raptor
  raptor_data_write8 : Raptor_lib/Data Storage/raptor_data_write  dataName='SWCU_BPSWU3_TEMP'  dataShape=Scalar  idxSource=Input Port  idxRow=1  idxCol=1
      settings: SourceProductName=Raptor
  raptor_data_write9 : Raptor_lib/Data Storage/raptor_data_write  dataName='SWCU_BPSWU3_VCELL_MAX'  dataShape=Scalar  idxSource=Input Port  idxRow=1  idxCol=1
      settings: SourceProductName=Raptor
  wires:
  raptor_can_rxmsg/3 -> raptor_data_write/1  "SWCU_BPSWU_HV_ENABLED"
  raptor_can_rxmsg/8 -> raptor_data_write6/1  "SWCU_BPSWU_CURR"
  raptor_can_rxmsg/6 -> raptor_data_write5/1  "SWCU_BPSWU_FCCAP"
  raptor_can_rxmsg/9 -> raptor_data_write7/1  "SWCU_BPSWU_VOLT"
  raptor_can_rxmsg/7 -> raptor_data_write4/1  "SWCU_BPSWU_RSOC"
  raptor_can_rxmsg/5 -> raptor_data_write3/1  "SWCU_BPSWU_EW_CODE"
  raptor_can_rxmsg/4 -> raptor_data_write2/1  "SWCU_BPSWU_EW"
  raptor_can_rxmsg/11 -> raptor_data_write9/1  "SWCU_BPSWU_VCELL_MAX"
  raptor_can_rxmsg/12 -> raptor_data_write10/1  "SWCU_BPSWU_VCELL_MIN"
  raptor_can_rxmsg/2 -> raptor_data_write1/1  "SWCU_BPSWU_READY"
  raptor_can_rxmsg/10 -> raptor_data_write8/1  "SWCU_BPSWU_TEMP"

== system EPT/Foreground_TimeBase_5ms/CHG//DCHG_PW_Control/CHG//DCHG_Current_Control/Idchg_con Soft Recovery/Delay1 ==
  Condition : Inport
  TimeCount : Inport  Port=2
  Constant10 : Constant
  Constant11 : Constant  Value=0
  Constant8 : Constant  Value=0
  CycleTrigger : Subsystem
  Switch2 : Switch  Threshold=1
  Switch3 : Switch  Threshold=1
  Unit Delay1 : UnitDelay  SampleTime=-1  HasFrameUpgradeWarning=on
  Unit Delay2 : UnitDelay  SampleTime=-1  HasFrameUpgradeWarning=on
  Output : Outport  VectorParamsAs1DForOutWhenUnconnected=off
  wires:
  Unit Delay1/1 -> Output/1
  Switch2/1 -> Unit Delay2/1
  Unit Delay2/1 -> Switch3/1
  Constant11/1 -> Switch3/3
  Switch3/1 -> CycleTrigger/1(In1)
  Constant10/1 -> Switch2/3
  Constant8/1 -> Switch2/1
  CycleTrigger/1(Trigger) -> Unit Delay1/1, Switch2/2
  Condition/1 -> Switch3/2
  TimeCount/1 -> CycleTrigger/2(In2)

== system EPT/Foreground_TimeBase_5ms/CHG//DCHG_PW_Control/CHG//DCHG_Current_Control/Idchg_con Soft Recovery/Latch1 ==
  Latch : Inport
  Reset : Inport  Port=2
  Switch1 : Switch  Criteria=u2 > Threshold
  Switch3 : Switch  Criteria=u2 > Threshold
  Unit Delay1 : UnitDelay  SampleTime=-1  HasFrameUpgradeWarning=on
  Output : Outport  VectorParamsAs1DForOutWhenUnconnected=off
  wires:
  Unit Delay1/1 -> Switch1/3
  Switch3/1 -> Output/1, Unit Delay1/1
  Reset/1 -> Switch3/2
  Latch/1 -> Switch1/1, Switch1/2
  Switch1/1 -> Switch3/3

== system EPT/Foreground_TimeBase_5ms/CHG//DCHG_PW_Control/CHG//DCHG_Current_Control/Idchg_con Soft Recovery /Delay1 ==
  Condition : Inport
  TimeCount : Inport  Port=2
  Constant10 : Constant
  Constant11 : Constant  Value=0
  Constant8 : Constant  Value=0
  CycleTrigger : Subsystem
  Switch2 : Switch  Threshold=1
  Switch3 : Switch  Threshold=1
  Unit Delay1 : UnitDelay  SampleTime=-1  HasFrameUpgradeWarning=on
  Unit Delay2 : UnitDelay  SampleTime=-1  HasFrameUpgradeWarning=on
  Output : Outport  VectorParamsAs1DForOutWhenUnconnected=off
  wires:
  Unit Delay1/1 -> Output/1
  Switch2/1 -> Unit Delay2/1
  Unit Delay2/1 -> Switch3/1
  Constant11/1 -> Switch3/3
  Switch3/1 -> CycleTrigger/1(In1)
  Constant10/1 -> Switch2/3
  Constant8/1 -> Switch2/1
  CycleTrigger/1(Trigger) -> Unit Delay1/1, Switch2/2
  Condition/1 -> Switch3/2
  TimeCount/1 -> CycleTrigger/2(In2)

== system EPT/Foreground_TimeBase_5ms/CHG//DCHG_PW_Control/CHG//DCHG_Current_Control/Idchg_con Soft Recovery /Latch1 ==
  Latch : Inport
  Reset : Inport  Port=2
  Switch1 : Switch  Criteria=u2 > Threshold
  Switch3 : Switch  Criteria=u2 > Threshold
  Unit Delay1 : UnitDelay  SampleTime=-1  HasFrameUpgradeWarning=on
  Output : Outport  VectorParamsAs1DForOutWhenUnconnected=off
  wires:
  Unit Delay1/1 -> Switch1/3
  Switch3/1 -> Output/1, Unit Delay1/1
  Reset/1 -> Switch3/2
  Latch/1 -> Switch1/1, Switch1/2
  Switch1/1 -> Switch3/3

== system EPT/Foreground_TimeBase_5ms/CHG//DCHG_PW_Control/CHG//DCHG_Current_Control/Soft Recovery/Subsystem2 ==
  Idchg_con : Inport
  Delta_Idchg : Inport  Port=2
  Recovery_Time_Ft : Inport  Port=3
  Enable : EnablePort
  Add2 : Sum
  Add3 : Sum
  Delay : Delay  DelayLength=1
  Gain1 : Gain  Gain=-(1/200)
  Product : Product
  Gain_Integral : Outport
  wires:
  Delay/1 -> Add3/1, Add2/2
  Gain1/1 -> Product/2
  Add2/1 -> Delay/1
  Add3/1 -> Gain_Integral/1
  Idchg_con/1 -> Add3/2
  Delta_Idchg/1 -> Gain1/1
  Product/1 -> Add2/1
  Recovery_Time_Ft/1 -> Product/1

== system EPT/Foreground_TimeBase_5ms/CHG//DCHG_PW_Control/Coulomb Counting Algorithm/Coulomb Counting Algorithm/20ms ==
  note: EOD correct SOH
  Ampere input : Inport
  RC input : Inport  Port=2
  Trigger : TriggerPort  VariantControl=Variant  PortDimensions=1
  Add1 : Sum  Inputs=+-
  Add2 : Sum
  Add3 : Sum
  Constant1 : Constant  Value=0
  Constant2 : Constant  Value=0
  Constant3 : Constant  Value=50
  Constant4 : Constant  Value=3600
  CountTrigger3 : Subsystem
  Delay : Delay  DelayLength=1
  Delay1 : Delay  DelayLength=1  InitialCondition=0
  Divide1 : Product  Inputs=*/
  Divide3 : Product  Inputs=*/
  Open Circuit Voltage Method : Subsystem
  Switch{1..8} (8 alike) : Switch  Criteria=u2 > Threshold
  raptor_adjustment1 : Raptor_lib/Data Storage/raptor_adjustment  paramName='Cal_OCV_Method'  nameSource=Parameter  initValue=0.00  dataType=double  storage=Calibration  calDispType=Number  calEnum={'False', 'True'}  calGain=1.0  calOffset=0.0  calMax=inf  calMin=-inf  calFormat='-1'  calUnit=''  calHelp=''  calAccess=1  calFunction=raptor_xcp_function(gcb)  calDispHeaders=off  calColHeaders={'Col1' 'Col2' 'Col3'}  calRowHeaders={'Row1' 'Row2' 'Row3'}
      settings: SourceProductName=Raptor
  raptor_data_read1 : Raptor_lib/Data Storage/raptor_data_read  dataName='EPT_BPOBU_FCCAP'  dataShape=Scalar  idxSource=Input  idxRow=1  idxCol=1
      settings: SourceProductName=Raptor
  raptor_data_read15 : Raptor_lib/Data Storage/raptor_data_read  dataName='Min_CellV'  dataShape=Scalar  idxSource=Input  idxRow=1  idxCol=1
      settings: SourceProductName=Raptor
  raptor_data_read18 : Raptor_lib/Data Storage/raptor_data_read  dataName='Warning_EndOfDischarge'  dataShape=Scalar  idxSource=Input  idxRow=1  idxCol=1
      settings: SourceProductName=Raptor
  raptor_data_read19 : Raptor_lib/Data Storage/raptor_data_read  dataName='Warning_EndOfCharge'  dataShape=Scalar  idxSource=Input  idxRow=1  idxCol=1
      settings: SourceProductName=Raptor
  raptor_data_read4 : Raptor_lib/Data Storage/raptor_data_read  dataName='EEPROM_FCCAP'  dataShape=Scalar  idxSource=Input  idxRow=1  idxCol=1
      settings: SourceProductName=Raptor
  raptor_data_write2 : Raptor_lib/Data Storage/raptor_data_write  dataName='EPT_BPOBU_FCCAP'  dataShape=Scalar  idxSource=Input Port  idxRow=1  idxCol=1
      settings: SourceProductName=Raptor
  raptor_data_write7 : Raptor_lib/Data Storage/raptor_data_write  dataName='EPT_BPOBU_RCAP'  dataShape=Scalar  idxSource=Input Port  idxRow=1  idxCol=1
      settings: SourceProductName=Raptor
  raptor_override : Raptor_lib/Data Storage/raptor_override  paramName='Cal_EPT_BPOBU_RCAP'  nameSource=Parameter  measurement=None  calDispType=Number  calEnum={'False', 'True'}  calGain=1.0  calOffset=0.0  calMax=inf  calMin=-inf  calFormat='-1'  calUnit=''  calHelp=''  calAccess=1  calFunction=[raptor_xcp_function(gcb) '|' raptor_get_param_eval(gcb, 'paramName') '_Override']
      settings: SourceProductName=Raptor
  raptor_override2 : Raptor_lib/Data Storage/raptor_override  paramName='Cal_EPT_BPOBU_FCCAP'  nameSource=Parameter  measurement=None  calDispType=Number  calEnum={'False', 'True'}  calGain=1.0  calOffset=0.0  calMax=inf  calMin=-inf  calFormat='-1'  calUnit=''  calHelp=''  calAccess=1  calFunction=[raptor_xcp_function(gcb) '|' raptor_get_param_eval(gcb, 'paramName') '_Override']
      settings: SourceProductName=Raptor
  wires:
  Ampere input/1 -> Divide3/1
  Divide3/1 -> Add2/1
  Switch2/1 -> Divide1/1
  Delay1/1 -> Add2/2
  Switch1/1 -> Delay1/1
  Add2/1 -> Switch1/3, Switch2/1
  CountTrigger3/1(Tirgger) -> Switch2/2, Switch1/2
  Constant4/1 -> Divide1/2
  Constant1/1 -> Switch2/3, Switch1/1
  Divide1/1 -> Add3/1
  Add3/1 -> Switch3/3
  RC input/1 -> Add3/2
  Constant3/1 -> Divide3/2, CountTrigger3/1(Counter)
  Open Circuit Voltage Method/1(RC Output) -> Switch3/1
  raptor_adjustment1/1 -> Switch3/2
  raptor_data_read15/1 -> Open Circuit Voltage Method/1(Vcell Input)
  Switch4/1 -> Switch8/3, Switch5/3
  raptor_data_read19/1 -> Switch6/2, Switch4/2
  Switch5/1 -> raptor_override/1
  raptor_data_read1/1 -> Switch6/3, Switch4/1
  Constant2/1 -> Switch5/1
  raptor_override/1 -> raptor_data_write7/1
  Switch3/1 -> Switch4/3, Switch6/1
  Add1/1 -> Switch7/1
  raptor_data_read18/1 -> Switch8/2, Switch7/2, Switch5/2
  raptor_data_read4/1 -> Add1/1
  Switch8/1 -> Delay/1
  Delay/1 -> Add1/2, Switch8/1
  Switch6/1 -> raptor_override2/1, Switch7/3
  raptor_override2/1 -> raptor_data_write2/1

== system EPT/Foreground_TimeBase_5ms/CHG//DCHG_PW_Control/Coulomb Counting Algorithm/Coulomb Counting Algorithm/CountTrigger ==
  Counter : Inport
  Constant1 : Constant  Value=0
  Constant3 : Constant
  CycleTrigger : Subsystem
  Switch : Switch  Threshold=1
  Unit Delay1 : UnitDelay  SampleTime=-1  HasFrameUpgradeWarning=on
  Unit Delay2 : UnitDelay  SampleTime=-1  HasFrameUpgradeWarning=on
  Tirgger : Outport  VectorParamsAs1DForOutWhenUnconnected=off
  wires:
  Unit Delay2/1 -> Tirgger/1
  Unit Delay1/1 -> CycleTrigger/1(In1)
  CycleTrigger/1(Trigger) -> Unit Delay2/1, Switch/2
  Counter/1 -> CycleTrigger/2(In2)
  Constant1/1 -> Switch/1
  Constant3/1 -> Switch/3
  Switch/1 -> Unit Delay1/1

== system EPT/Foreground_TimeBase_5ms/CHG//DCHG_PW_Control/Coulomb Counting Algorithm/Delay/CycleTrigger ==
  In1 : Inport
  In2 : Inport  Port=2
  Add : Sum
  Add2 : Sum  Inputs=+-
  Constant2 : Constant  Value=0
  Constant3 : Constant
  Data Type Conversion1 : DataTypeConversion
  Data Type Conversion2 : DataTypeConversion
  Relational Operator1 : RelationalOperator  OutDataTypeStr=boolean  RndMeth=Simplest
  Saturation : Saturate  UpperLimit=inf  LowerLimit=2
  Switch : Switch  Threshold=1
  Unit Delay : UnitDelay  SampleTime=-1  HasFrameUpgradeWarning=on
  Trigger : Outport  VectorParamsAs1DForOutWhenUnconnected=off
  wires:
  Saturation/1 -> Add2/1
  Add/1 -> Switch/1
  In1/1 -> Data Type Conversion2/1
  Unit Delay/1 -> Add/1
  Switch/1 -> Relational Operator1/1, Unit Delay/1
  Relational Operator1/1 -> Trigger/1
  Data Type Conversion1/1 -> Relational Operator1/2
  Constant2/1 -> Switch/3
  Data Type Conversion2/1 -> Add/2, Switch/2
  Add2/1 -> Data Type Conversion1/1
  In2/1 -> Saturation/1
  Constant3/1 -> Add2/2

== system EPT/Foreground_TimeBase_5ms/CHG//DCHG_PW_Control/Coulomb Counting Algorithm/WH /20ms ==
  Ampere input : Inport
  Voltage input : Inport  Port=2
  WH Input : Inport  Port=3
  Trigger : TriggerPort  VariantControl=Variant  PortDimensions=1
  Add2 : Sum
  Add3 : Sum
  Constant1 : Constant  Value=0
  Constant3 : Constant  Value=50
  Constant4 : Constant  Value=3600
  CountTrigger3 : Subsystem
  Delay1 : Delay  DelayLength=1  InitialCondition=0
  Divide1 : Product  Inputs=*/
  Divide2 : Product  Inputs=**
  Divide3 : Product  Inputs=*/
  Switch1 : Switch  Criteria=u2 > Threshold
  Switch2 : Switch  Criteria=u2 > Threshold
  WH Output : Outport  VectorParamsAs1DForOutWhenUnconnected=off
  wires:
  Constant3/1 -> CountTrigger3/1(Counter), Divide3/2
  Add3/1 -> WH Output/1
  Divide1/1 -> Add3/1
  Constant1/1 -> Switch2/3, Switch1/1
  Constant4/1 -> Divide1/2
  CountTrigger3/1(Tirgger) -> Switch1/2, Switch2/2
  Add2/1 -> Switch2/1, Switch1/3
  Switch1/1 -> Delay1/1
  Delay1/1 -> Add2/2
  Switch2/1 -> Divide1/1
  Divide3/1 -> Add2/1
  Divide2/1 -> Divide3/1
  Ampere input/1 -> Divide2/1
  Voltage input/1 -> Divide2/2
  WH Input/1 -> Add3/2

== system EPT/Foreground_TimeBase_5ms/CHG//DCHG_PW_Control/Coulomb Counting Algorithm/WH /CountTrigger ==
  Counter : Inport
  Constant1 : Constant  Value=0
  Constant3 : Constant
  CycleTrigger : Subsystem
  Switch : Switch  Threshold=1
  Unit Delay1 : UnitDelay  SampleTime=-1  HasFrameUpgradeWarning=on
  Unit Delay2 : UnitDelay  SampleTime=-1  HasFrameUpgradeWarning=on
  Tirgger : Outport  VectorParamsAs1DForOutWhenUnconnected=off
  wires:
  Switch/1 -> Unit Delay1/1
  Constant3/1 -> Switch/3
  Constant1/1 -> Switch/1
  Counter/1 -> CycleTrigger/2(In2)
  CycleTrigger/1(Trigger) -> Switch/2, Unit Delay2/1
  Unit Delay1/1 -> CycleTrigger/1(In1)
  Unit Delay2/1 -> Tirgger/1
